simulink model "TerrainSimRunner"  (R2021a)
settings: Solver=VariableStepAuto  StartTime=0.0  StopTime=100  RelTol=1e-3
values from neighbouring files (symbols this model uses):
  init_parameters = struct    [TerrainGenerator.m]    (also in init_parameters.mat = )
undefined symbols (not defined in the file or in its folder): r0, x0, y0
libraries: vrlib x3
settings Model: Creator=16109  LastModifiedBy=16109

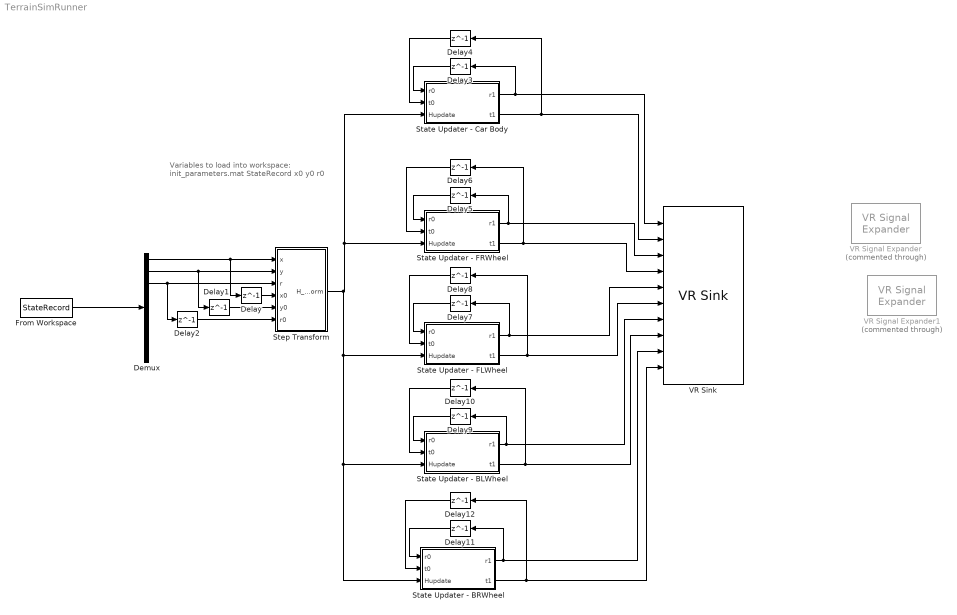
== system TerrainSimRunner ==
  note: Variables to load into workspace:
      | init_parameters.mat
      | StateRecord
      | x0
      | y0
      | r0
  Delay : Delay  DelayLength=1  InitialCondition=x0
  Delay1 : Delay  DelayLength=1  InitialCondition=y0
  Delay10 : Delay  DelayLength=1  InitialCondition=init_parameters.BLTranslation
  Delay11 : Delay  DelayLength=1  InitialCondition=init_parameters.BRRotation
  Delay12 : Delay  DelayLength=1  InitialCondition=init_parameters.BLTranslation
  Delay2 : Delay  DelayLength=1  InitialCondition=r0
  Delay3 : Delay  DelayLength=1  InitialCondition=init_parameters.BodyRotation
  Delay4 : Delay  DelayLength=1  InitialCondition=init_parameters.BodyTranslation
  Delay5 : Delay  DelayLength=1  InitialCondition=init_parameters.FRWheelRotation
  Delay6 : Delay  DelayLength=1  InitialCondition=init_parameters.FRWheelTranslation
  Delay7 : Delay  DelayLength=1  InitialCondition=init_parameters.FLWheelRotation
  Delay8 : Delay  DelayLength=1  InitialCondition=init_parameters.FLWheelTranslation
  Delay9 : Delay  DelayLength=1  InitialCondition=init_parameters.BLRotation
  Demux : Demux  Outputs=9
  From Workspace : FromWorkspace  VariableName=StateRecord
  State Updater - BLWheel : MATLAB Function  TreatAsAtomicUnit=on
  State Updater - BRWheel : MATLAB Function  TreatAsAtomicUnit=on
  State Updater - Car Body : MATLAB Function  TreatAsAtomicUnit=on
  State Updater - FLWheel : MATLAB Function  TreatAsAtomicUnit=on
  State Updater - FRWheel : MATLAB Function  TreatAsAtomicUnit=on
  Step Transform : MATLAB Function  TreatAsAtomicUnit=on
  VR Signal Expander : vrlib/VR Signal Expander  Commented=through  outwidth=4  outidx=[2 4]
  VR Signal Expander1 : vrlib/VR Signal Expander  Commented=through  outwidth=3  outidx=[1]
  VR Sink : vrlib/VR Sink  InstantiateOnLoad=on  SampleTime=0.1  ViewEnable=on  RemoteChange=off  RemoteView=off  FieldsWritten=CarBody.rotation.4.1.1.double#CarBody.translation.3.1.1.double#FRWheel.rotation.4.1.1.double#FRWheel.translation.3.1.1.double#FLWheel.rotation.4.1.1.double#FLWheel.translation.3.1.1.double#BLWheel.rotation.4.1.1.double#BLWheel.translation.3.1.1.double#BRWheel.rotation.4.1.1.double#BRWheel.translation.3.1.1.double  WorldFileName=TerrainSimulation.x3d  AutoView=off  VideoDimensions=[]  AllowVariableSize=off
  wires:
  From Workspace/1 -> Demux/1
  Demux/1 -> Delay/1, Step Transform/1(x)
  Demux/2 -> Delay1/1, Step Transform/2(y)
  Demux/3 -> Delay2/1, Step Transform/3(r)
  Delay/1 -> Step Transform/4(x0)
  Delay1/1 -> Step Transform/5(y0)
  Delay2/1 -> Step Transform/6(r0)
  Step Transform/1(H_transform) -> State Updater - BRWheel/3(Hupdate), State Updater - BLWheel/3(Hupdate), State Updater - FLWheel/3(Hupdate), State Updater - FRWheel/3(Hupdate), State Updater - Car Body/3(Hupdate)
  State Updater - Car Body/1(r1) -> Delay3/1, VR Sink/1
  State Updater - Car Body/2(t1) -> Delay4/1, VR Sink/2
  State Updater - FRWheel/1(r1) -> Delay5/1, VR Sink/3
  State Updater - FRWheel/2(t1) -> Delay6/1, VR Sink/4
  State Updater - FLWheel/1(r1) -> Delay7/1, VR Sink/5
  State Updater - FLWheel/2(t1) -> Delay8/1, VR Sink/6
  State Updater - BLWheel/1(r1) -> Delay9/1, VR Sink/7
  State Updater - BLWheel/2(t1) -> Delay10/1, VR Sink/8
  State Updater - BRWheel/1(r1) -> Delay11/1, VR Sink/9
  State Updater - BRWheel/2(t1) -> Delay12/1, VR Sink/10
  Delay3/1 -> State Updater - Car Body/1(r0)
  Delay4/1 -> State Updater - Car Body/2(t0)
  Delay5/1 -> State Updater - FRWheel/1(r0)
  Delay6/1 -> State Updater - FRWheel/2(t0)
  Delay7/1 -> State Updater - FLWheel/1(r0)
  Delay8/1 -> State Updater - FLWheel/2(t0)
  Delay9/1 -> State Updater - BLWheel/1(r0)
  Delay10/1 -> State Updater - BLWheel/2(t0)
  Delay11/1 -> State Updater - BRWheel/1(r0)
  Delay12/1 -> State Updater - BRWheel/2(t0)

== matlab function TerrainSimRunner/State Updater - Car Body ==
  data: r0 input; t0 input; r1 output; Hupdate input; t1 output
function [r1, t1]= fcn(r0, t0,Hupdate)
r0_matrix = axang2rotm(r0);
t0 = [t0; 0];
H0 = [r0_matrix, t0; 0 ,0, 0 , 1];
H1 = Hupdate * H0;
r1 = rotm2axang(H1(1:3,1:3));
t1 = H0(1:3,4);
end

== matlab function TerrainSimRunner/Step Transform ==
  data: x input; H_transform output; y input; r input; x0 input; y0 input; r0 input
function H_transform = fcn(x, y, r, x0, y0, r0)
H_transform = [
    cos(r-r0), -sin(r-r0), 0, x-x0;
    sin(r-r0), cos(r-r0), 0, y-y0;
    0, 0, 1, 0
    0, 0, 0, 1];
end

== matlab function TerrainSimRunner/State Updater - FRWheel ==
  data: r0 input; t0 input; r1 output; Hupdate input; t1 output
function [r1, t1]= fcn(r0, t0,Hupdate)
r0_matrix = axang2rotm(r0);
t0 = [t0; 0];
H0 = [r0_matrix, t0; 0 ,0, 0 , 1];
H1 = Hupdate * H0;
r1 = rotm2axang(H1(1:3,1:3));
t1 = H0(1:3,4);
end

== matlab function TerrainSimRunner/State Updater - FLWheel ==
  data: r0 input; t0 input; r1 output; Hupdate input; t1 output
function [r1, t1]= fcn(r0, t0,Hupdate)
r0_matrix = axang2rotm(r0);
t0 = [t0; 0];
H0 = [r0_matrix, t0; 0 ,0, 0 , 1];
H1 = Hupdate * H0;
r1 = rotm2axang(H1(1:3,1:3));
t1 = H0(1:3,4);
end

== matlab function TerrainSimRunner/State Updater - BLWheel ==
  data: r0 input; t0 input; r1 output; Hupdate input; t1 output
function [r1, t1]= fcn(r0, t0,Hupdate)
r0_matrix = axang2rotm(r0);
t0 = [t0; 0];
H0 = [r0_matrix, t0; 0 ,0, 0 , 1];
H1 = Hupdate * H0;
r1 = rotm2axang(H1(1:3,1:3));
t1 = H0(1:3,4);
end

== matlab function TerrainSimRunner/State Updater - BRWheel ==
  data: r0 input; t0 input; r1 output; Hupdate input; t1 output
function [r1, t1]= fcn(r0, t0,Hupdate)
r0_matrix = axang2rotm(r0);
t0 = [t0; 0];
H0 = [r0_matrix, t0; 0 ,0, 0 , 1];
H1 = Hupdate * H0;
r1 = rotm2axang(H1(1:3,1:3));
t1 = H0(1:3,4);
end
